simulink library "idealSensors_cl"  (R2020a)
settings: Solver=VariableStepAuto  StartTime=0.0  StopTime=10.0  RelTol=1e-3
undefined symbols (not defined in the file or in its folder): initializeBussesFromBlock
settings Model: Creator=mcobb  LastModifiedBy=John Jr
settings DataIOCC: ReturnWorkspaceOutputs=off
settings DebuggingCC: ArithmeticOperatorsInVariantConditions=warning
settings SFSimCC: CustomCodeUndefinedFunction=UseInterfaceOnly

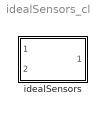
== system idealSensors_cl ==
  idealSensors : Subsystem  LoadFcn=initializeBussesFromBlock(gcb)  InitFcn=initializeBussesFromBlock(gcb)  StartFcn=initializeBussesFromBlock(gcb)

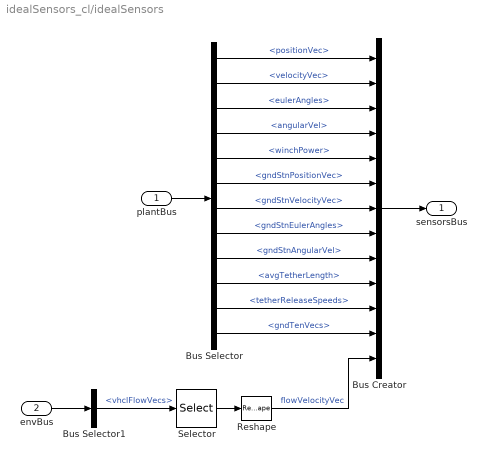
== system idealSensors_cl/idealSensors ==
  plantBus : Inport  OutDataTypeStr=Bus: plantBus
  envBus : Inport  Port=2  OutDataTypeStr=Bus: envBus
  Bus Creator : BusCreator  Inputs=13  OutDataTypeStr=Bus: sensorsBus  NonVirtualBus=on
  Bus Selector : BusSelector  OutputSignals=positionVec,velocityVec,eulerAngles,angularVel,winchPower,gndStnPositionVec,gndStnVelocityVec,gndStnEulerAngles,gndStnAngularVel,avgTetherLength,tetherReleaseSpeeds,gndTenVecs
  Bus Selector1 : BusSelector  OutputSignals=vhclFlowVecs
  Reshape : Reshape  OutputDimensionality=Column vector (2-D)
  Selector : Selector  NumberOfDimensions=2  InputPortWidth=3  IndexOptions=Select all,Index vector (dialog)  Indices=[1 3],1  OutputSizes=1,1
  sensorsBus : Outport  OutDataTypeStr=Bus: sensorsBus  VectorParamsAs1DForOutWhenUnconnected=off
  wires:
  plantBus/1 -> Bus Selector/1
  envBus/1 -> Bus Selector1/1
  Bus Selector1/1 -> Selector/1  "<vhclFlowVecs>"
  Selector/1 -> Reshape/1
  Reshape/1 -> Bus Creator/13  "flowVelocityVec"
  Bus Creator/1 -> sensorsBus/1
  Bus Selector/1 -> Bus Creator/1  "<positionVec>"
  Bus Selector/12 -> Bus Creator/12  "<gndTenVecs>"
  Bus Selector/2 -> Bus Creator/2  "<velocityVec>"
  Bus Selector/3 -> Bus Creator/3  "<eulerAngles>"
  Bus Selector/4 -> Bus Creator/4  "<angularVel>"
  Bus Selector/5 -> Bus Creator/5  "<winchPower>"
  Bus Selector/6 -> Bus Creator/6  "<gndStnPositionVec>"
  Bus Selector/7 -> Bus Creator/7  "<gndStnVelocityVec>"
  Bus Selector/8 -> Bus Creator/8  "<gndStnEulerAngles>"
  Bus Selector/9 -> Bus Creator/9  "<gndStnAngularVel>"
  Bus Selector/10 -> Bus Creator/10  "<avgTetherLength>"
  Bus Selector/11 -> Bus Creator/11  "<tetherReleaseSpeeds>"
